simulink subsystem "AC_tank_R2024a"  (R2024a)
settings: Solver=VariableStepAuto  StartTime=0.0  StopTime=10.0  RelTol=1e-3
undefined symbols (not defined in the file or in its folder): AC_tank_weight, Ambient_temp, Initial_temp
libraries: fl_lib x5, nesl_utility x2, SimscapeFluids_lib x1
settings Model: Creator=MW  LastModifiedBy=MW

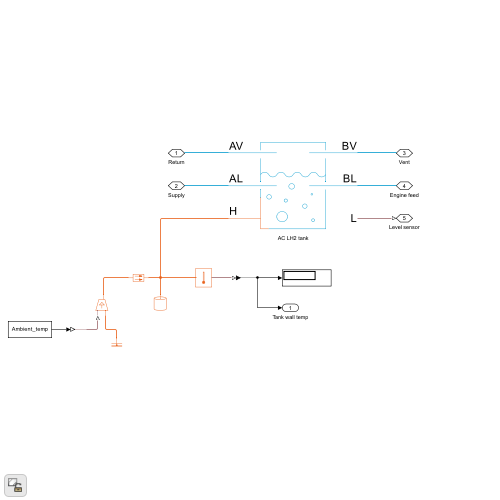
[thumbnail: Simulink's stored preview of the top-level diagram]
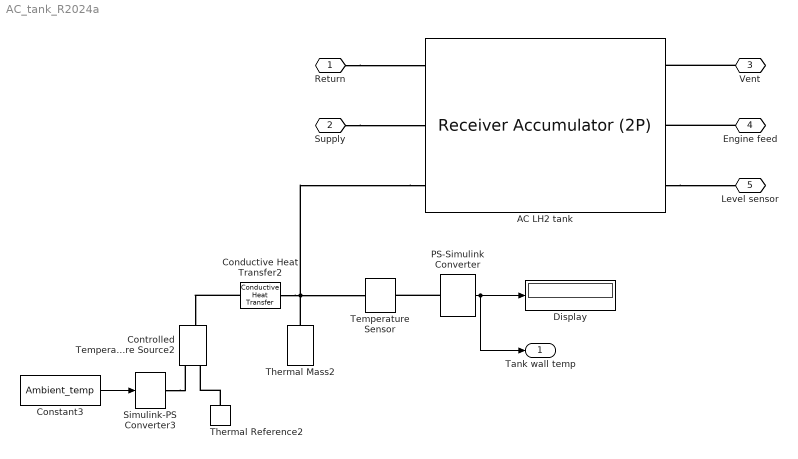
== system AC_tank_R2024a ==
  AC LH2 tank : SimscapeFluids_lib/Two-Phase Fluid/Tanks & Accumulators/Receiver Accumulator (2P)  volume=AC_tank_volume m^3  tank_area=AC_tank_cross_sectional_area m^2  area_AV=AC_return_line_port_inner_area m^2  area_BV=return_pipe_inner_area m^2  area_AL=AC_supply_line_port_inner_area m^2  area_BL=AC_engine_feed_port_inner_area m^2  V_frac_liq_error=simscape.enum.assert.action.none  V_frac_liq_min=0.05  V_frac_liq_max=0.95  V_frac_smooth=0.01  p_crit_error=simscape.enum.assert.action.error  hc_vap=AC_tank_vapour_heat_transfer_coeff W/(K*m^2)  hc_liq=AC_tank_liquid_heat_transfer_coeff W/(K*m^2)  p_init=Initial_AC_tank_pressure bar  fraction_spec=fluids.two_phase_fluid.tanks_accumulators.enum.LiquidFractionSpec.Volume  M_frac_liq_init=0.5  V_frac_liq_init=Initial_AC_LH2_frac  saturated_init=false  energy_spec=fluids.two_phase_fluid.tanks_accumulators.enum.EnergySpec.Temperature  delta_T_sub_init=5 deltaK  delta_T_sup_init=5 deltaK  T_liq_init=Initial_AC_Tank_Liquid_Temp K  T_vap_init=Initial_AC_Tank_Gas_Temp K  h_liq_init=400 kJ/kg  h_vap_init=2700 kJ/kg  u_liq_init=400 kJ/kg  u_vap_init=2700 kJ/kg  tau_vap_cond=0.1 s
      settings: InternalSimscapePortConfiguration="{\"Bottom\":[],\"Left\":[{\"id\":\"AV\",\"label\":\"AV\",\"type\":\"foundation.two_phase_fluid.two_phase_fluid\"},{\"id\":\"AL\",\"label\":\"AL\",\"type\":\"foundation.two_phase_fluid.two_phase_fluid\"},{\"id\":\"H\",\"label\":\"H\",\"type\":\"foundation.thermal.thermal\"}],\"Right\":[{\"id\":\"BV\",\"label\":\"BV\",\"type\":\"foundation.two_phase_fluid.two_phase_fluid\"},{\"id\":\"BL\",\"label\":\"BL\",\"type\":\"foundation.two_phase_fluid.two_phase_fluid\"},{\"id\":\"L\",\"label\":\"L\",\"type\":\"output\"}],\"Top\":[]}"
  Conductive Heat Transfer2 : fl_lib/Thermal/Thermal Elements/Conductive Heat Transfer  thermal_type=foundation.enum.ConstantVariableTabulated.Constant  wall_geometry=foundation.enum.ConductionWallGeometry.Planar  area=AC_tank_surface_area m^2  thickness=AC_wall_thickness m  d_in=0.05 m  d_out=0.1 m  L=1 m  th_cond_min=10 W/(K*m)  th_cond=0.001 W/(m*K)  th_cond_TLU=[413, 401, 392, 383, 371, 357, 342] W/(K*m)  temp_TLU=[200, 273, 400, 600, 800, 1000, 1200] K  T_specify=off  T_priority=None  T=0 K  T_nominal_specify=off  T_nominal_value=1  T_nominal_unit=K  Q_specify=off  Q_priority=None  Q=0 W  Q_nominal_specify=off  Q_nominal_value=1  Q_nominal_unit=W
  Constant3 : Constant  Value=Ambient_temp
  Controlled Temperature Source2 : fl_lib/Thermal/Thermal Sources/Controlled Temperature Source
  Display : Display
  PS-Simulink Converter : nesl_utility/PS-Simulink Converter  PhysicalDomain=network_engine_domain  SubClassName=ps_output  LeftPortType=input  RightPortType=output  PseudoPeriodic=off  Frequencies=[]  VectorFormat=inherit  Unit=inherit  AffineConversion=off
  Simulink-PS Converter3 : nesl_utility/Simulink-PS Converter  PhysicalDomain=network_engine_domain  SubClassName=ps_input  LeftPortType=input  RightPortType=output  PseudoPeriodic=off  Frequencies=[]  NoiseDistribution=none  NoiseParameters=[]  Unit=1  AffineConversion=off  FilteringAndDerivatives=zero  SimscapeFilterOrder=1  InputFilterTimeConstant=0.001  UdotUserProvided=1
  Temperature Sensor : fl_lib/Thermal/Thermal Sensors/Temperature Sensor  temperature_measure=foundation.enum.MeasurementReference.absolute
      settings: InternalSimscapePortConfiguration="{\"Bottom\":[],\"Left\":[{\"id\":\"A\",\"label\":\"A\",\"type\":\"foundation.thermal.thermal\"}],\"Right\":[{\"id\":\"T\",\"label\":\"T\",\"type\":\"output\"}],\"Top\":[]}"
  Thermal Mass2 : fl_lib/Thermal/Thermal Elements/Thermal Mass  mass_type=foundation.enum.constant_variable.constant  mass=AC_tank_weight/2 kg  sp_heat=250 J/kg/K  mass_min=1e-6 kg  num_ports=foundation.enum.numPorts2.one  m_specify=off  m_priority=High  m=1 kg  m_nominal_specify=off  m_nominal_value=1  m_nominal_unit=kg  T_specify=on  T_priority=High  T=Initial_temp K  T_nominal_specify=off  T_nominal_value=1  T_nominal_unit=K  Q_specify=off  Q_priority=None  Q=0 W  Q_nominal_specify=off  Q_nominal_value=1  Q_nominal_unit=W
  Thermal Reference2 : fl_lib/Thermal/Thermal Elements/Thermal Reference
  Return : PMIOPort  Side=Left
  Supply : PMIOPort  Port=2  Side=Left
  Vent : PMIOPort  Port=3  Side=Right
  Engine feed : PMIOPort  Port=4  Side=Right
  Level sensor : PMIOPort  Port=5  Side=Right
  Tank wall temp : Outport
  wires:
  PS-Simulink Converter/1 -> Tank wall temp/1, Display/1
  Constant3/1 -> Simulink-PS Converter3/1
  connections:
  AC LH2 tank/LConn3 -- Conductive Heat Transfer2/RConn1 -- Thermal Mass2/LConn1 -- Temperature Sensor/LConn1
  PS-Simulink Converter/LConn1 -- Temperature Sensor/RConn1
  AC LH2 tank/RConn3 -- Level sensor/RConn1
  Engine feed/RConn1 -- AC LH2 tank/RConn2
  Vent/RConn1 -- AC LH2 tank/RConn1
  Return/RConn1 -- AC LH2 tank/LConn1
  Supply/RConn1 -- AC LH2 tank/LConn2
  Thermal Reference2/LConn1 -- Controlled Temperature Source2/RConn2
  Simulink-PS Converter3/RConn1 -- Controlled Temperature Source2/RConn1
  Conductive Heat Transfer2/LConn1 -- Controlled Temperature Source2/LConn1
